simulink model "MultipleAgentsChoice_NoVR"  (Simulink 7.5)
settings: Solver=ode45  StartTime=0.0  StopTime=1000  RelTol=1e-4  AbsTol=1e-4
libraries: simulink x64
(part 3 of 6)

== system MultipleAgentsChoice_NoVR/StatePropagation/SatelliteControlAccel/Agent Body1/Actual Thruster response ==
  note: RELIABLE THRUSTER?
  Signals : Inport  OutDataType=sfix(16)  OutScaling=2^0
  AgentNumber : Inport  Port=2  OutDataType=sfix(16)  OutScaling=2^0
  Bus Creator{,1..3} (4 alike) : BusCreator  Inputs=3
  Bus Creator4 : BusCreator
  Bus Selector : BusSelector  OutputSignals=A1ControlSignals,ConfigurationSignals.XValves1,ConfigurationSignals.XSwitch1,ConfigurationSignals.YValves,ConfigurationSignals.YSwitch,ConfigurationSignals.ZValves,ConfigurationSignals.ZSwitch,ConfigurationSignals.XYZValves,ConfigurationSignals.XYZSwitch,ConfigurationSignals.A1Break
  Bus Selector1 : BusSelector  OutputSignals=signal1.L1Vent,signal1.L2Vent,signal2.L1Vent,signal2.L2Vent,signal3.L1Vent,signal3.L2Vent,XYZ.L1Vent,XYZ.L2Vent  OutputAsBus=on
  Constant{,1..3} (4 alike) : Constant  OutDataType=sfix(16)  OutScaling=2^0
  Conv2XYZ : MATLABFcn  MATLABFcn=Conv2XYZ_multi  OutputDimensions=3
  Demux : Demux
  Derivative : Derivative
  Mux : Mux  Inputs=5
  Mux1 : Mux  Inputs=2
  PressureTank : Subsystem
  Reliable : Constant  OutDataType=sfix(16)  OutScaling=2^0
  Sum : Sum  Inputs=|++  OutDataType=sfix(16)  OutScaling=2^0
  Switch : simulink/Signal Routing/Manual Switch  SystemSampleTime=-1  sw=1  action=0  varsize=off
  ThrusterSuiteNumber1 : Constant  Value=4  OutDataType=sfix(16)  OutScaling=2^0
  Unreliable : Constant  Value=0  OutDataType=sfix(16)  OutScaling=2^0
  VentForce : MATLABFcn  MATLABFcn=VentForce_multi  OutputDimensions=3
  XYZthruster : Subsystem
  Xthruster : Subsystem
  Ythruster1 : Subsystem
  Zthruster1 : Subsystem
  XThrusterData : Outport  OutDataType=sfix(16)  OutScaling=2^0
  YThrusterData : Outport  Port=2  OutDataType=sfix(16)  OutScaling=2^0
  ZThrusterData : Outport  Port=3  OutDataType=sfix(16)  OutScaling=2^0
  XYZThrusterData : Outport  Port=4  OutDataType=sfix(16)  OutScaling=2^0
  Forces : Outport  Port=5  OutDataType=sfix(16)  OutScaling=2^0
  PressureData : Outport  Port=6  OutDataType=sfix(16)  OutScaling=2^0
  wires:
  Bus Selector/9 -> Bus Creator3/3  "<XYZSwitch>"
  Bus Selector/8 -> Bus Creator3/2  "<XYZValves>"
  Bus Creator3/1 -> XYZthruster/3(Data)
  Constant2/1 -> Bus Creator3/1
  Demux/4 -> XYZthruster/2(ForceRequest)
  XYZthruster/2(XYZforces) -> Mux/4
  XYZthruster/1(XYZData) -> XYZThrusterData/1  "A1XYZThrusterData"
  Bus Selector/4 -> Bus Creator1/2  "<YValves>"
  Zthruster1/2(Zforces) -> Mux/3
  Bus Creator2/1 -> Zthruster1/3(Data)
  Constant1/1 -> Bus Creator2/1
  Bus Creator1/1 -> Ythruster1/3(Data)
  Constant/1 -> Bus Creator1/1
  Bus Selector/3 -> Bus Creator/3  "<XSwitch1>"
  Bus Selector/2 -> Bus Creator/2  "<XValves1>"
  Bus Creator/1 -> Xthruster/3(Data)
  Zthruster1/1(ZData) -> ZThrusterData/1  "A1ZThrusterData"
  Ythruster1/1(YData) -> YThrusterData/1  "A1YThrusterData"
  Xthruster/1(XData) -> XThrusterData/1
  Ythruster1/2(Yforces) -> Mux/2
  Demux/3 -> Zthruster1/2(ForceRequest)
  Demux/2 -> Ythruster1/2(ForceRequest)
  Bus Selector/7 -> Bus Creator2/3  "<ZSwitch>"
  Bus Selector/6 -> Bus Creator2/2  "<ZValves>"
  Bus Selector/5 -> Bus Creator1/3  "<YSwitch>"
  Xthruster/2(Xforces) -> Mux/1
  Demux/1 -> Xthruster/2(ForceRequest)
  Bus Selector/1 -> Demux/1  "<A1ControlSignals>"
  Mux/1 -> Conv2XYZ/1
  Signals/1 -> Bus Selector/1
  Constant3/1 -> Bus Creator/1
  AgentNumber/1 -> Mux/5
  Mux1/1 -> PressureData/1
  Bus Creator4/1 -> PressureTank/2(GroupVentData), Bus Selector1/1
  PressureTank/1(TankPressure) -> [FeedPressure], Derivative/1, Mux1/1  "MainTankPressure"
  ThrusterSuiteNumber1/1 -> [NumThrusters]
  [VentY] -> Bus Creator4/2
  [VentZ] -> Bus Creator4/3
  [VentXYZ] -> Bus Creator4/4
  [VentX] -> Bus Creator4/1
  Xthruster/3(ActivityData) -> [VentX]
  XYZthruster/3(Activitydata) -> [VentXYZ]
  Zthruster1/3(Activitydata) -> [VentZ]
  Ythruster1/3(ActivityData) -> [VentY]
  [FeedPressure] -> Xthruster/1(FeedPressure)
  [FeedPressure] -> Ythruster1/1(FeedPressure)
  [FeedPressure] -> Zthruster1/1(FeedPressure)
  [FeedPressure] -> XYZthruster/1(FeedPressure)
  [NumThrusters] -> PressureTank/1(NumThrusters)
  Derivative/1 -> Mux1/2  "MainTankDerrivative"
  Switch/1 -> Zthruster1/4(Reliability)
  Reliable/1 -> Switch/1
  Unreliable/1 -> Switch/2
  Bus Selector/10 -> Zthruster1/5(BrokenLine)  "<A1Break>"
  Conv2XYZ/1 -> Sum/2
  VentForce/1 -> Sum/1
  Sum/1 -> Forces/1
  Bus Selector1/1 -> VentForce/1

== system MultipleAgentsChoice_NoVR/StatePropagation/SatelliteControlAccel/Agent Body1/Convert2Accels ==
  note: convert forces to accelerations based on 20kg mass and conv to km units
  Forces : Inport  OutDataType=sfix(16)  OutScaling=2^0
  Conv KM : Gain  Gain=0.001  ParameterDataType=sfix(16)  ParameterScaling=2^0  OutDataType=sfix(16)  OutScaling=2^0
  mass : Gain  Gain=0.05  ParameterDataType=sfix(16)  ParameterScaling=2^0  OutDataType=sfix(16)  OutScaling=2^0
  Accels : Outport  OutDataType=sfix(16)  OutScaling=2^0
  wires:
  Forces/1 -> mass/1
  Conv KM/1 -> Accels/1
  mass/1 -> Conv KM/1

== system MultipleAgentsChoice_NoVR/StatePropagation/SatelliteControlAccel/Agent Body2/Actual Thruster response ==
  note: UNRELIABLE THRUSTER?
  Signals : Inport  OutDataType=sfix(16)  OutScaling=2^0
  AgentNumber : Inport  Port=2  OutDataType=sfix(16)  OutScaling=2^0
  Bus Creator{,1..3} (4 alike) : BusCreator  Inputs=3
  Bus Creator4 : BusCreator
  Bus Selector : BusSelector  OutputSignals=A2ControlSignals,ConfigurationSignals.XValves1,ConfigurationSignals.XSwitch1,ConfigurationSignals.YValves,ConfigurationSignals.YSwitch,ConfigurationSignals.ZValves,ConfigurationSignals.ZSwitch,ConfigurationSignals.XYZValves,ConfigurationSignals.XYZSwitch,ConfigurationSignals.A2Break
  Bus Selector1 : BusSelector  OutputSignals=signal1.L1Vent,signal1.L2Vent,signal2.L1Vent,signal2.L2Vent,signal3.L1Vent,signal3.L2Vent,XYZ.L1Vent,XYZ.L2Vent  OutputAsBus=on
  Constant{,1..3} (4 alike) : Constant  OutDataType=sfix(16)  OutScaling=2^0
  Conv2XYZ : MATLABFcn  MATLABFcn=Conv2XYZ_multi  OutputDimensions=3
  Demux : Demux
  Derivative : Derivative
  Mux : Mux  Inputs=5
  Mux1 : Mux  Inputs=2
  PressureTank : Subsystem
  Reliable : Constant  OutDataType=sfix(16)  OutScaling=2^0
  Sum : Sum  Inputs=|++  OutDataType=sfix(16)  OutScaling=2^0
  Switch : simulink/Signal Routing/Manual Switch  SystemSampleTime=-1  sw=1  action=0  varsize=off
  ThrusterSuiteNumber1 : Constant  Value=4  OutDataType=sfix(16)  OutScaling=2^0
  Unreliable : Constant  Value=0  OutDataType=sfix(16)  OutScaling=2^0
  VentForce : MATLABFcn  MATLABFcn=VentForce_multi  OutputDimensions=3
  XYZthruster : Subsystem
  Xthruster : Subsystem
  Ythruster1 : Subsystem
  Zthruster1 : Subsystem
  XThrusterData : Outport  OutDataType=sfix(16)  OutScaling=2^0
  YThrusterData : Outport  Port=2  OutDataType=sfix(16)  OutScaling=2^0
  ZThrusterData : Outport  Port=3  OutDataType=sfix(16)  OutScaling=2^0
  XYZThrusterData : Outport  Port=4  OutDataType=sfix(16)  OutScaling=2^0
  Forces : Outport  Port=5  OutDataType=sfix(16)  OutScaling=2^0
  PressureData : Outport  Port=6  OutDataType=sfix(16)  OutScaling=2^0
  wires:
  Derivative/1 -> Mux1/2  "MainTankDerrivative"
  [NumThrusters] -> PressureTank/1(NumThrusters)
  [FeedPressure] -> XYZthruster/1(FeedPressure)
  [FeedPressure] -> Zthruster1/1(FeedPressure)
  [FeedPressure] -> Ythruster1/1(FeedPressure)
  [FeedPressure] -> Xthruster/1(FeedPressure)
  Ythruster1/3(ActivityData) -> [VentY]
  Zthruster1/3(Activitydata) -> [VentZ]
  XYZthruster/3(Activitydata) -> [VentXYZ]
  Xthruster/3(ActivityData) -> [VentX]
  [VentX] -> Bus Creator4/1
  [VentXYZ] -> Bus Creator4/4
  [VentZ] -> Bus Creator4/3
  [VentY] -> Bus Creator4/2
  ThrusterSuiteNumber1/1 -> [NumThrusters]
  PressureTank/1(TankPressure) -> Mux1/1, Derivative/1, [FeedPressure]  "MainTankPressure"
  Bus Creator4/1 -> PressureTank/2(GroupVentData), Bus Selector1/1
  Mux1/1 -> PressureData/1
  AgentNumber/1 -> Mux/5
  Constant3/1 -> Bus Creator/1
  Signals/1 -> Bus Selector/1
  Mux/1 -> Conv2XYZ/1
  Bus Selector/1 -> Demux/1  "<A2ControlSignals>"
  Demux/1 -> Xthruster/2(ForceRequest)
  Xthruster/2(Xforces) -> Mux/1
  Bus Selector/5 -> Bus Creator1/3  "<YSwitch>"
  Bus Selector/6 -> Bus Creator2/2  "<ZValves>"
  Bus Selector/7 -> Bus Creator2/3  "<ZSwitch>"
  Demux/2 -> Ythruster1/2(ForceRequest)
  Demux/3 -> Zthruster1/2(ForceRequest)
  Ythruster1/2(Yforces) -> Mux/2
  Xthruster/1(XData) -> XThrusterData/1  "A2XThrusterData"
  Ythruster1/1(YData) -> YThrusterData/1  "A2YThrusterData"
  Zthruster1/1(ZData) -> ZThrusterData/1  "A2ZThrusterData"
  Bus Creator/1 -> Xthruster/3(Data)
  Bus Selector/2 -> Bus Creator/2  "<XValves1>"
  Bus Selector/3 -> Bus Creator/3  "<XSwitch1>"
  Constant/1 -> Bus Creator1/1
  Bus Creator1/1 -> Ythruster1/3(Data)
  Constant1/1 -> Bus Creator2/1
  Bus Creator2/1 -> Zthruster1/3(Data)
  Zthruster1/2(Zforces) -> Mux/3
  Bus Selector/4 -> Bus Creator1/2  "<YValves>"
  XYZthruster/1(XYZData) -> XYZThrusterData/1  "A2XYZThrusterData"
  XYZthruster/2(XYZforces) -> Mux/4
  Demux/4 -> XYZthruster/2(ForceRequest)
  Constant2/1 -> Bus Creator3/1
  Bus Creator3/1 -> XYZthruster/3(Data)
  Bus Selector/8 -> Bus Creator3/2  "<XYZValves>"
  Bus Selector/9 -> Bus Creator3/3  "<XYZSwitch>"
  Unreliable/1 -> Switch/2
  Reliable/1 -> Switch/1
  Switch/1 -> Zthruster1/4(Reliability)
  Bus Selector/10 -> Zthruster1/5(BrokenLine)  "<A2Break>"
  VentForce/1 -> Sum/1
  Sum/1 -> Forces/1
  Conv2XYZ/1 -> Sum/2
  Bus Selector1/1 -> VentForce/1

== system MultipleAgentsChoice_NoVR/StatePropagation/SatelliteControlAccel/Agent Body2/Convert2Accels ==
  note: convert forces to accelerations based on 20kg mass and conv to km units
  Forces : Inport  OutDataType=sfix(16)  OutScaling=2^0
  Conv KM : Gain  Gain=0.001  ParameterDataType=sfix(16)  ParameterScaling=2^0  OutDataType=sfix(16)  OutScaling=2^0
  mass : Gain  Gain=0.05  ParameterDataType=sfix(16)  ParameterScaling=2^0  OutDataType=sfix(16)  OutScaling=2^0
  Accels : Outport  OutDataType=sfix(16)  OutScaling=2^0
  wires:
  mass/1 -> Conv KM/1
  Conv KM/1 -> Accels/1
  Forces/1 -> mass/1

== system MultipleAgentsChoice_NoVR/StatePropagation/SatelliteControlAccel/Agent Body3/Actual Thruster response ==
  note: UNRELIABLE THRUSTER?
  Signals : Inport  OutDataType=sfix(16)  OutScaling=2^0
  AgentNumber : Inport  Port=2  OutDataType=sfix(16)  OutScaling=2^0
  Bus Creator{,1..3} (4 alike) : BusCreator  Inputs=3
  Bus Creator4 : BusCreator
  Bus Selector : BusSelector  OutputSignals=A3ControlSignals,ConfigurationSignals.XValves1,ConfigurationSignals.XSwitch1,ConfigurationSignals.YValves,ConfigurationSignals.YSwitch,ConfigurationSignals.ZValves,ConfigurationSignals.ZSwitch,ConfigurationSignals.XYZValves,ConfigurationSignals.XYZSwitch,ConfigurationSignals.A3Break
  Bus Selector1 : BusSelector  OutputSignals=signal1.L1Vent,signal1.L2Vent,signal2.L1Vent,signal2.L2Vent,signal3.L1Vent,signal3.L2Vent,XYZ.L1Vent,XYZ.L2Vent  OutputAsBus=on
  Constant{,1..3} (4 alike) : Constant  OutDataType=sfix(16)  OutScaling=2^0
  Conv2XYZ : MATLABFcn  MATLABFcn=Conv2XYZ_multi  OutputDimensions=3
  Demux : Demux
  Derivative : Derivative
  Mux : Mux  Inputs=5
  Mux1 : Mux  Inputs=2
  PressureTank : Subsystem
  Reliable : Constant  OutDataType=sfix(16)  OutScaling=2^0
  Sum : Sum  Inputs=|++  OutDataType=sfix(16)  OutScaling=2^0
  Switch : simulink/Signal Routing/Manual Switch  SystemSampleTime=-1  sw=1  action=0  varsize=off
  ThrusterSuiteNumber1 : Constant  Value=4  OutDataType=sfix(16)  OutScaling=2^0
  Unreliable : Constant  Value=0  OutDataType=sfix(16)  OutScaling=2^0
  VentForce : MATLABFcn  MATLABFcn=VentForce_multi  OutputDimensions=3
  XYZthruster : Subsystem
  Xthruster : Subsystem
  Ythruster1 : Subsystem
  Zthruster1 : Subsystem
  XThrusterData : Outport  OutDataType=sfix(16)  OutScaling=2^0
  YThrusterData : Outport  Port=2  OutDataType=sfix(16)  OutScaling=2^0
  ZThrusterData : Outport  Port=3  OutDataType=sfix(16)  OutScaling=2^0
  XYZThrusterData : Outport  Port=4  OutDataType=sfix(16)  OutScaling=2^0
  Forces : Outport  Port=5  OutDataType=sfix(16)  OutScaling=2^0
  PressureData : Outport  Port=6  OutDataType=sfix(16)  OutScaling=2^0
  wires:
  Derivative/1 -> Mux1/2  "MainTankDerrivative"
  [NumThrusters] -> PressureTank/1(NumThrusters)
  [FeedPressure] -> XYZthruster/1(FeedPressure)
  [FeedPressure] -> Zthruster1/1(FeedPressure)
  [FeedPressure] -> Ythruster1/1(FeedPressure)
  [FeedPressure] -> Xthruster/1(FeedPressure)
  Ythruster1/3(ActivityData) -> [VentY]
  Zthruster1/3(Activitydata) -> [VentZ]
  XYZthruster/3(Activitydata) -> [VentXYZ]
  Xthruster/3(ActivityData) -> [VentX]
  [VentX] -> Bus Creator4/1
  [VentXYZ] -> Bus Creator4/4
  [VentZ] -> Bus Creator4/3
  [VentY] -> Bus Creator4/2
  ThrusterSuiteNumber1/1 -> [NumThrusters]
  PressureTank/1(TankPressure) -> Mux1/1, Derivative/1, [FeedPressure]  "MainTankPressure"
  Bus Creator4/1 -> PressureTank/2(GroupVentData), Bus Selector1/1
  Mux1/1 -> PressureData/1
  AgentNumber/1 -> Mux/5
  Constant3/1 -> Bus Creator/1
  Signals/1 -> Bus Selector/1
  Mux/1 -> Conv2XYZ/1
  Bus Selector/1 -> Demux/1  "<A3ControlSignals>"
  Demux/1 -> Xthruster/2(ForceRequest)
  Xthruster/2(Xforces) -> Mux/1
  Bus Selector/5 -> Bus Creator1/3  "<YSwitch>"
  Bus Selector/6 -> Bus Creator2/2  "<ZValves>"
  Bus Selector/7 -> Bus Creator2/3  "<ZSwitch>"
  Demux/2 -> Ythruster1/2(ForceRequest)
  Demux/3 -> Zthruster1/2(ForceRequest)
  Ythruster1/2(Yforces) -> Mux/2
  Xthruster/1(XData) -> XThrusterData/1  "A3XThrusterData"
  Ythruster1/1(YData) -> YThrusterData/1  "A3YThrusterData"
  Zthruster1/1(ZData) -> ZThrusterData/1  "A3ZThrusterData"
  Bus Creator/1 -> Xthruster/3(Data)
  Bus Selector/2 -> Bus Creator/2  "<XValves1>"
  Bus Selector/3 -> Bus Creator/3  "<XSwitch1>"
  Constant/1 -> Bus Creator1/1
  Bus Creator1/1 -> Ythruster1/3(Data)
  Constant1/1 -> Bus Creator2/1
  Bus Creator2/1 -> Zthruster1/3(Data)
  Zthruster1/2(Zforces) -> Mux/3
  Bus Selector/4 -> Bus Creator1/2  "<YValves>"
  XYZthruster/1(XYZData) -> XYZThrusterData/1  "A3XYZThrusterData"
  XYZthruster/2(XYZforces) -> Mux/4
  Demux/4 -> XYZthruster/2(ForceRequest)
  Constant2/1 -> Bus Creator3/1
  Bus Creator3/1 -> XYZthruster/3(Data)
  Bus Selector/8 -> Bus Creator3/2  "<XYZValves>"
  Bus Selector/9 -> Bus Creator3/3  "<XYZSwitch>"
  Unreliable/1 -> Switch/2
  Reliable/1 -> Switch/1
  Switch/1 -> Zthruster1/4(Reliability)
  Bus Selector/10 -> Zthruster1/5(BrokenLine)  "<A3Break>"
  VentForce/1 -> Sum/1
  Sum/1 -> Forces/1
  Conv2XYZ/1 -> Sum/2
  Bus Selector1/1 -> VentForce/1

== system MultipleAgentsChoice_NoVR/StatePropagation/SatelliteControlAccel/Agent Body3/Convert2Accels ==
  note: convert forces to accelerations based on 20kg mass and conv to km units
  Forces : Inport  OutDataType=sfix(16)  OutScaling=2^0
  Conv KM : Gain  Gain=0.001  ParameterDataType=sfix(16)  ParameterScaling=2^0  OutDataType=sfix(16)  OutScaling=2^0
  mass : Gain  Gain=0.05  ParameterDataType=sfix(16)  ParameterScaling=2^0  OutDataType=sfix(16)  OutScaling=2^0
  Accels : Outport  OutDataType=sfix(16)  OutScaling=2^0
  wires:
  Forces/1 -> mass/1
  Conv KM/1 -> Accels/1
  mass/1 -> Conv KM/1

== system MultipleAgentsChoice_NoVR/StatePropagation/SatelliteControlAccel/GetCmdAIL/Triggered run ==
  Trigger : TriggerPort
  DimentionsOut1 : Constant  Value=127  OutDataType=sfix(16)  OutScaling=2^0
  GetCmdAILXYZ : MATLABFcn  MATLABFcn=GetCmdAIL  OutputDimensions=127
  Commands : Outport  OutDataType=sfix(16)  OutScaling=2^0
  wires:
  DimentionsOut1/1 -> GetCmdAILXYZ/1
  GetCmdAILXYZ/1 -> Commands/1

== system MultipleAgentsChoice_NoVR/StatePropagation/SatelliteControlAccel/Selective Hill State Provision and Discretisation/Agent1 ==
  GEOC_Current : Inport  OutDataType=sfix(16)  OutScaling=2^0
  LeadAgent : Inport  Port=2  OutDataType=sfix(16)  OutScaling=2^0
  Bus Creator : BusCreator  Inputs=5
  Bus Selector2 : BusSelector  OutputSignals=Agent1Pos,Agent1Vel,Agent2Pos,Agent2Vel,Agent3Pos,Agent3Vel
  Demux : Demux  Outputs=7
  Hill State multi : MATLABFcn  MATLABFcn=HillErrors_multi  OutputDimensions=7
  Multiport Switch : MultiPortSwitch  zeroidx=off
  Mux1 : Mux  Inputs=3
  Mux2 : Mux  Inputs=3
  Mux{3..6} (4 alike) : Mux  Inputs=2
  Zero-Order Hold3 : ZeroOrderHold  SampleTime=0.5
  Zero-Order Hold4 : ZeroOrderHold  SampleTime=0.5
  Agent1 : Outport  OutDataType=sfix(16)  OutScaling=2^0
  wires:
  Mux1/1 -> Zero-Order Hold4/1, Bus Creator/3  "HillVelCont"
  Mux2/1 -> Zero-Order Hold3/1, Bus Creator/2  "HillPosCont"
  Demux/2 -> Mux2/1
  Demux/4 -> Mux2/3
  Demux/3 -> Mux2/2
  Demux/7 -> Mux1/3
  Demux/5 -> Mux1/1
  Demux/6 -> Mux1/2
  Hill State multi/1 -> Demux/1
  LeadAgent/1 -> Multiport Switch/1
  GEOC_Current/1 -> Bus Selector2/1
  Demux/1 -> Bus Creator/1  "HillMagCont"
  Bus Creator/1 -> Agent1/1  "A1HillState"
  Mux3/1 -> Hill State multi/1
  Bus Selector2/1 -> Mux4/1  "<Agent1Pos>"
  Bus Selector2/2 -> Mux4/2  "<Agent1Vel>"
  Bus Selector2/3 -> Mux5/1  "<Agent2Pos>"
  Bus Selector2/4 -> Mux5/2  "<Agent2Vel>"
  Bus Selector2/5 -> Mux6/1  "<Agent3Pos>"
  Bus Selector2/6 -> Mux6/2  "<Agent3Vel>"
  Mux4/1 -> [Agent1]
  Mux5/1 -> [Agent2]
  Mux6/1 -> [Agent3]
  Multiport Switch/1 -> Mux3/2
  [Agent1] -> Multiport Switch/2
  [Agent2] -> Multiport Switch/3
  [Agent3] -> Multiport Switch/4
  [Agent1] -> Mux3/1
  Zero-Order Hold4/1 -> Bus Creator/5  "HillVelDisc"
  Zero-Order Hold3/1 -> Bus Creator/4  "HillPosDisc"

== system MultipleAgentsChoice_NoVR/StatePropagation/SatelliteControlAccel/Selective Hill State Provision and Discretisation/Agent2 ==
  GEOC_Current : Inport  OutDataType=sfix(16)  OutScaling=2^0
  LeadAgent : Inport  Port=2  OutDataType=sfix(16)  OutScaling=2^0
  Bus Creator : BusCreator  Inputs=5
  Bus Selector2 : BusSelector  OutputSignals=Agent1Pos,Agent1Vel,Agent2Pos,Agent2Vel,Agent3Pos,Agent3Vel
  Demux : Demux  Outputs=7
  Hill State multi : MATLABFcn  MATLABFcn=HillErrors_multi  OutputDimensions=7
  Multiport Switch : MultiPortSwitch  zeroidx=off
  Mux1 : Mux  Inputs=3
  Mux2 : Mux  Inputs=3
  Mux{3..6} (4 alike) : Mux  Inputs=2
  Zero-Order Hold3 : ZeroOrderHold  SampleTime=0.5
  Zero-Order Hold4 : ZeroOrderHold  SampleTime=0.5
  Agent2 : Outport  OutDataType=sfix(16)  OutScaling=2^0
  wires:
  [Agent3] -> Multiport Switch/4
  [Agent2] -> Multiport Switch/3
  [Agent1] -> Multiport Switch/2
  Multiport Switch/1 -> Mux3/2
  Mux6/1 -> [Agent3]
  Mux5/1 -> [Agent2]
  Mux4/1 -> [Agent1]
  Bus Selector2/6 -> Mux6/2  "<Agent3Vel>"
  Bus Selector2/5 -> Mux6/1  "<Agent3Pos>"
  Bus Selector2/4 -> Mux5/2  "<Agent2Vel>"
  Bus Selector2/3 -> Mux5/1  "<Agent2Pos>"
  Bus Selector2/2 -> Mux4/2  "<Agent1Vel>"
  Bus Selector2/1 -> Mux4/1  "<Agent1Pos>"
  [Agent2] -> Mux3/1
  Mux3/1 -> Hill State multi/1
  Bus Creator/1 -> Agent2/1  "A2HillState"
  Demux/1 -> Bus Creator/1  "HillMagCont"
  GEOC_Current/1 -> Bus Selector2/1
  LeadAgent/1 -> Multiport Switch/1
  Hill State multi/1 -> Demux/1
  Demux/6 -> Mux1/2
  Demux/5 -> Mux1/1
  Demux/7 -> Mux1/3
  Demux/3 -> Mux2/2
  Demux/4 -> Mux2/3
  Demux/2 -> Mux2/1
  Mux2/1 -> Zero-Order Hold3/1, Bus Creator/2  "HillPosCont"
  Mux1/1 -> Zero-Order Hold4/1, Bus Creator/3  "HillVelCont"
  Zero-Order Hold3/1 -> Bus Creator/4  "HillPosDisc"
  Zero-Order Hold4/1 -> Bus Creator/5  "HillVelDisc"

== system MultipleAgentsChoice_NoVR/StatePropagation/SatelliteControlAccel/Selective Hill State Provision and Discretisation/Agent3 ==
  GEOC_Current : Inport  OutDataType=sfix(16)  OutScaling=2^0
  LeadAgent : Inport  Port=2  OutDataType=sfix(16)  OutScaling=2^0
  Bus Creator : BusCreator  Inputs=5
  Bus Selector2 : BusSelector  OutputSignals=Agent1Pos,Agent1Vel,Agent2Pos,Agent2Vel,Agent3Pos,Agent3Vel
  Demux : Demux  Outputs=7
  Hill State multi : MATLABFcn  MATLABFcn=HillErrors_multi  OutputDimensions=7
  Multiport Switch : MultiPortSwitch  zeroidx=off
  Mux1 : Mux  Inputs=3
  Mux2 : Mux  Inputs=3
  Mux{3..6} (4 alike) : Mux  Inputs=2
  Zero-Order Hold3 : ZeroOrderHold  SampleTime=0.5
  Zero-Order Hold4 : ZeroOrderHold  SampleTime=0.5
  Agent3 : Outport  OutDataType=sfix(16)  OutScaling=2^0
  wires:
  Mux1/1 -> Zero-Order Hold4/1, Bus Creator/3  "HillVelCont"
  Mux2/1 -> Zero-Order Hold3/1, Bus Creator/2  "HillPosCont"
  Demux/2 -> Mux2/1
  Demux/4 -> Mux2/3
  Demux/3 -> Mux2/2
  Demux/7 -> Mux1/3
  Demux/5 -> Mux1/1
  Demux/6 -> Mux1/2
  Hill State multi/1 -> Demux/1
  LeadAgent/1 -> Multiport Switch/1
  GEOC_Current/1 -> Bus Selector2/1
  Zero-Order Hold4/1 -> Bus Creator/5  "HillVelDisc"
  Demux/1 -> Bus Creator/1  "HillMagCont"
  Bus Creator/1 -> Agent3/1  "A3HillState"
  Mux3/1 -> Hill State multi/1
  Bus Selector2/1 -> Mux4/1  "<Agent1Pos>"
  Bus Selector2/2 -> Mux4/2  "<Agent1Vel>"
  Bus Selector2/3 -> Mux5/1  "<Agent2Pos>"
  Bus Selector2/4 -> Mux5/2  "<Agent2Vel>"
  Bus Selector2/5 -> Mux6/1  "<Agent3Pos>"
  Bus Selector2/6 -> Mux6/2  "<Agent3Vel>"
  Mux4/1 -> [Agent1]
  Mux5/1 -> [Agent2]
  Mux6/1 -> [Agent3]
  [Agent1] -> Multiport Switch/2
  [Agent2] -> Multiport Switch/3
  [Agent3] -> Multiport Switch/4
  [Agent3] -> Mux3/1
  Multiport Switch/1 -> Mux3/2
  Zero-Order Hold3/1 -> Bus Creator/4  "HillPosDisc"

== system MultipleAgentsChoice_NoVR/StatePropagation/SatelliteControlAccel/Selective Hill State Provision and Discretisation/MemoryUpdate ==
  GEOC_Current : Inport  OutDataType=sfix(16)  OutScaling=2^0
  LeadAgent : Inport  Port=2  OutDataType=sfix(16)  OutScaling=2^0
  Bus Selector2 : BusSelector  OutputSignals=Agent1Pos,Agent1Vel,Agent2Pos,Agent2Vel,Agent3Pos,Agent3Vel
  Multiport Switch : MultiPortSwitch  zeroidx=off
  Mux4 : Mux  Inputs=2
  Mux5 : Mux  Inputs=2
  Mux6 : Mux  Inputs=2
  Updatememory : MATLABFcn  MATLABFcn=UpdateMemory  OutputDimensions=0
  wires:
  Multiport Switch/1 -> Updatememory/1
  Mux6/1 -> Multiport Switch/4
  Mux5/1 -> Multiport Switch/3
  Mux4/1 -> Multiport Switch/2
  Bus Selector2/6 -> Mux6/2  "<Agent3Vel>"
  Bus Selector2/5 -> Mux6/1  "<Agent3Pos>"
  Bus Selector2/4 -> Mux5/2  "<Agent2Vel>"
  Bus Selector2/3 -> Mux5/1  "<Agent2Pos>"
  Bus Selector2/2 -> Mux4/2  "<Agent1Vel>"
  Bus Selector2/1 -> Mux4/1  "<Agent1Pos>"
  GEOC_Current/1 -> Bus Selector2/1
  LeadAgent/1 -> Multiport Switch/1

== system MultipleAgentsChoice_NoVR/StatePropagation/SatelliteControlAccel/TriggeredSendAgent/SendToAIL ==
  A1ActualForces : Inport  OutDataType=sfix(16)  OutScaling=2^0
  A1PlanMsg : Inport  Port=2  OutDataType=sfix(16)  OutScaling=2^0
  A1DesiredForces : Inport  Port=3  OutDataType=sfix(16)  OutScaling=2^0
  A1StateInfo : Inport  Port=4  OutDataType=sfix(16)  OutScaling=2^0
  A1tank : Inport  Port=5  OutDataType=sfix(16)  OutScaling=2^0
  A1XThruster : Inport  Port=6  OutDataType=sfix(16)  OutScaling=2^0
  A1YThruster : Inport  Port=7  OutDataType=sfix(16)  OutScaling=2^0
  A1ZThruster : Inport  Port=8  OutDataType=sfix(16)  OutScaling=2^0
  A1XYZThruster : Inport  Port=9  OutDataType=sfix(16)  OutScaling=2^0
  A2ActualForces : Inport  Port=10  OutDataType=sfix(16)  OutScaling=2^0
  A2PlanMsg : Inport  Port=11  OutDataType=sfix(16)  OutScaling=2^0
  A2DesiredForces : Inport  Port=12  OutDataType=sfix(16)  OutScaling=2^0
  A2StateInfo : Inport  Port=13  OutDataType=sfix(16)  OutScaling=2^0
  A2tank : Inport  Port=14  OutDataType=sfix(16)  OutScaling=2^0
  A2XThruster : Inport  Port=15  OutDataType=sfix(16)  OutScaling=2^0
  A2YThruster : Inport  Port=16  OutDataType=sfix(16)  OutScaling=2^0
  A2ZThruster : Inport  Port=17  OutDataType=sfix(16)  OutScaling=2^0
  A2XYZThruster : Inport  Port=18  OutDataType=sfix(16)  OutScaling=2^0
  A3ActualForces : Inport  Port=19  OutDataType=sfix(16)  OutScaling=2^0
  A3PlanMsg : Inport  Port=20  OutDataType=sfix(16)  OutScaling=2^0
  A3DesiredForces : Inport  Port=21  OutDataType=sfix(16)  OutScaling=2^0
  A3StateInfo : Inport  Port=22  OutDataType=sfix(16)  OutScaling=2^0
  A3tank : Inport  Port=23  OutDataType=sfix(16)  OutScaling=2^0
  A3XThruster : Inport  Port=24  OutDataType=sfix(16)  OutScaling=2^0
  A3YThruster : Inport  Port=25  OutDataType=sfix(16)  OutScaling=2^0
  A3ZThruster : Inport  Port=26  OutDataType=sfix(16)  OutScaling=2^0
  A3XYZThruster : Inport  Port=27  OutDataType=sfix(16)  OutScaling=2^0
  Display : Display
  MATLAB Fcn : MATLABFcn  MATLABFcn=CommunicateWithTagsMulti  OutputDimensions=0
  Mux : Mux  Inputs=27
  wires:
  A1ActualForces/1 -> Mux/1  "A1ActualForces"
  A1PlanMsg/1 -> Mux/2  "A1PlanMsg"
  A1StateInfo/1 -> Mux/4  "A1StateInfo"
  A1XThruster/1 -> Mux/6  "A1XThruster"
  A1YThruster/1 -> Mux/7  "A1YThruster"
  A1ZThruster/1 -> Mux/8  "A1ZThruster"
  A1DesiredForces/1 -> Mux/3  "A1DesiredForfces"
  A1tank/1 -> Mux/5  "A1Tank"
  A2ActualForces/1 -> Mux/10  "A2ActualForces"
  A2PlanMsg/1 -> Mux/11  "A2PlanMsg"
  A2StateInfo/1 -> Mux/13  "A2StateInfo"
  A2XThruster/1 -> Mux/15  "A2XThruster"
  A2YThruster/1 -> Mux/16  "A2YThruster"
  A2ZThruster/1 -> Mux/17  "A2ZThruster"
  A2DesiredForces/1 -> Mux/12  "A2DesiredForces"
  A2tank/1 -> Mux/14  "A2Tank"
  A1XYZThruster/1 -> Mux/9  "A1XYZThruster"
  A2XYZThruster/1 -> Mux/18  "A2XYZThruster"
  A3PlanMsg/1 -> Mux/20  "A3PlanMsg"
  A3DesiredForces/1 -> Mux/21  "A3DesiredForces"
  A3StateInfo/1 -> Mux/22  "A3StateInfo"
  A3tank/1 -> Mux/23  "A3Tank"
  A3XThruster/1 -> Mux/24  "A3XThruster"
  A3YThruster/1 -> Mux/25  "A3YThruster"
  A3ZThruster/1 -> Mux/26  "A3ZThruster"
  A3XYZThruster/1 -> Mux/27  "A3XYZThruster"
  A3ActualForces/1 -> Mux/19  "A3ActualForces"
  Mux/1 -> MATLAB Fcn/1, Display/1

== system MultipleAgentsChoice_NoVR/StatePropagation/SatelliteControlAccel/TriggeredSendCont/SendToCont ==
  A1ActualForces : Inport  OutDataType=sfix(16)  OutScaling=2^0
  A1PlanMsg : Inport  Port=2  OutDataType=sfix(16)  OutScaling=2^0
  A1DesiredForces : Inport  Port=3  OutDataType=sfix(16)  OutScaling=2^0
  A1StateInfo : Inport  Port=4  OutDataType=sfix(16)  OutScaling=2^0
  A1tank : Inport  Port=5  OutDataType=sfix(16)  OutScaling=2^0
  A1XThruster : Inport  Port=6  OutDataType=sfix(16)  OutScaling=2^0
  A1YThruster : Inport  Port=7  OutDataType=sfix(16)  OutScaling=2^0
  A1ZThruster : Inport  Port=8  OutDataType=sfix(16)  OutScaling=2^0
  A1XYZThruster : Inport  Port=9  OutDataType=sfix(16)  OutScaling=2^0
  A2ActualForces : Inport  Port=10  OutDataType=sfix(16)  OutScaling=2^0
  A2PlanMsg : Inport  Port=11  OutDataType=sfix(16)  OutScaling=2^0
  A2DesiredForces : Inport  Port=12  OutDataType=sfix(16)  OutScaling=2^0
  A2StateInfo : Inport  Port=13  OutDataType=sfix(16)  OutScaling=2^0
  A2tank : Inport  Port=14  OutDataType=sfix(16)  OutScaling=2^0
  A2XThruster : Inport  Port=15  OutDataType=sfix(16)  OutScaling=2^0
  A2YThruster : Inport  Port=16  OutDataType=sfix(16)  OutScaling=2^0
  A2ZThruster : Inport  Port=17  OutDataType=sfix(16)  OutScaling=2^0
  A2XYZThruster : Inport  Port=18  OutDataType=sfix(16)  OutScaling=2^0
  A3ActualForces : Inport  Port=19  OutDataType=sfix(16)  OutScaling=2^0
  A3PlanMsg : Inport  Port=20  OutDataType=sfix(16)  OutScaling=2^0
  A3DesiredForces : Inport  Port=21  OutDataType=sfix(16)  OutScaling=2^0
  A3StateInfo : Inport  Port=22  OutDataType=sfix(16)  OutScaling=2^0
  A3tank : Inport  Port=23  OutDataType=sfix(16)  OutScaling=2^0
  A3XThruster : Inport  Port=24  OutDataType=sfix(16)  OutScaling=2^0
  A3YThruster : Inport  Port=25  OutDataType=sfix(16)  OutScaling=2^0
  A3ZThruster : Inport  Port=26  OutDataType=sfix(16)  OutScaling=2^0
  A3XYZThruster : Inport  Port=27  OutDataType=sfix(16)  OutScaling=2^0
  Display : Display
  MATLAB Fcn : MATLABFcn  MATLABFcn=CommunicateWithCont  OutputDimensions=0
  Mux : Mux  Inputs=27
  wires:
  Mux/1 -> Display/1, MATLAB Fcn/1
  A3ActualForces/1 -> Mux/19  "A3ActualForces"
  A3XYZThruster/1 -> Mux/27  "A3XYZThruster"
  A3ZThruster/1 -> Mux/26  "A3ZThruster"
  A3YThruster/1 -> Mux/25  "A3YThruster"
  A3XThruster/1 -> Mux/24  "A3XThruster"
  A3tank/1 -> Mux/23  "A3tank"
  A3StateInfo/1 -> Mux/22  "A3StateInfo"
  A3DesiredForces/1 -> Mux/21  "A3DesiredForces"
  A3PlanMsg/1 -> Mux/20  "A3PlanMsg"
  A2XYZThruster/1 -> Mux/18  "A2XYZThruster"
  A1XYZThruster/1 -> Mux/9  "A1XYZThruster"
  A2tank/1 -> Mux/14  "A2tank"
  A2DesiredForces/1 -> Mux/12  "A2DesiredForces"
  A2ZThruster/1 -> Mux/17  "A2ZThruster"
  A2YThruster/1 -> Mux/16  "A2YThruster"
  A2XThruster/1 -> Mux/15  "A2XThruster"
  A2StateInfo/1 -> Mux/13  "A2StateInfo"
  A2PlanMsg/1 -> Mux/11  "A2PlanMsg"
  A2ActualForces/1 -> Mux/10  "A2ActualForces"
  A1tank/1 -> Mux/5  "A1tank"
  A1DesiredForces/1 -> Mux/3  "A1DesiredForfces"
  A1ZThruster/1 -> Mux/8  "A1ZThruster"
  A1YThruster/1 -> Mux/7  "A1YThruster"
  A1XThruster/1 -> Mux/6  "A1XThruster"
  A1StateInfo/1 -> Mux/4  "A1StateInfo"
  A1PlanMsg/1 -> Mux/2  "A1PlanMsg"
  A1ActualForces/1 -> Mux/1  "A1ActualForces"

== system MultipleAgentsChoice_NoVR/StatePropagation/SatelliteControlAccel/Agent Body1/Actual Thruster response/PressureTank ==
  NumThrusters : Inport  OutDataType=sfix(16)  OutScaling=2^0
  GroupVentData : Inport  Port=2  OutDataType=sfix(16)  OutScaling=2^0
  Clock : Clock
      settings: Decimation=10
  Display : Display
  DropRate : MATLABFcn  MATLABFcn=DropRate_multi  OutputDimensions=1
  Integrator : Integrator  InitialConditionSource=external
  Mux : Mux  Inputs=2
  Start : Constant  Value=0  OutDataType=sfix(16)  OutScaling=2^0
  StartPressure : Constant  Value=100  OutDataType=sfix(16)  OutScaling=2^0
  Switch1 : Switch
  TankPressure : Outport  OutDataType=sfix(16)  OutScaling=2^0
  wires:
  DropRate/1 -> Switch1/1
  Mux/1 -> DropRate/1
  NumThrusters/1 -> Mux/1
  GroupVentData/1 -> Mux/2
  Switch1/1 -> Integrator/1
  Clock/1 -> Switch1/2
  Start/1 -> Switch1/3
  Integrator/1 -> Display/1, TankPressure/1
  StartPressure/1 -> Integrator/2

== system MultipleAgentsChoice_NoVR/StatePropagation/SatelliteControlAccel/Agent Body1/Actual Thruster response/XYZthruster ==
  note: NB:-Agent has no knowledge of red blocks
      |             -Blue blocks prescribed by agent
  note: Tank pressure and thruster selection: must declare number of thrusters
  FeedPressure : Inport  OutDataType=sfix(16)  OutScaling=2^0
  ForceRequest : Inport  Port=2  OutDataType=sfix(16)  OutScaling=2^0
  Data : Inport  Port=3  OutDataType=sfix(16)  OutScaling=2^0
  Bus Creator2 : BusCreator  Inputs=3
  Bus Selector : BusSelector  OutputSignals=XYZValves,XYZSwitch
  Constant : Constant  OutDataType=sfix(16)  OutScaling=2^0
  Constant1 : Constant  Value=0  OutDataType=sfix(16)  OutScaling=2^0
  Switch : Switch  Criteria=u2 ~= 0
  Thruster1 : Subsystem
  XYZData : Outport  OutDataType=sfix(16)  OutScaling=2^0
  XYZforces : Outport  Port=2  OutDataType=sfix(16)  OutScaling=2^0
  Activitydata : Outport  Port=3  OutDataType=sfix(16)  OutScaling=2^0
  wires:
  ForceRequest/1 -> Thruster1/4(ForceRequest)  "XYZforces"
  Thruster1/1(L1Vent) -> Bus Creator2/1  "L1Vent"
  Thruster1/2(L2Vent) -> Bus Creator2/2  "L2Vent"
  FeedPressure/1 -> Thruster1/2(FeedPressure)
  Constant/1 -> Switch/1
  Constant1/1 -> Switch/3
  Thruster1/4(thrusterData) -> XYZData/1  "A1TXYZ1"
  Data/1 -> Bus Selector/1
  Bus Selector/1 -> Thruster1/1(ValveAssign)  "<XYZValves>"
  Bus Selector/2 -> Thruster1/3(MainSwitch)  "<XYZSwitch>"
  Thruster1/3(Forces) -> XYZforces/1, Switch/2
  Switch/1 -> Bus Creator2/3  "Active1"
  Bus Creator2/1 -> Activitydata/1  "XYZ"

== system MultipleAgentsChoice_NoVR/StatePropagation/SatelliteControlAccel/Agent Body1/Actual Thruster response/Xthruster ==
  note: Tank pressure and thruster selection: must declare number of thrusters
  note: NB:-Agent has no knowledge of red blocks
      |             -Blue blocks prescribed by agent
  FeedPressure : Inport  OutDataType=sfix(16)  OutScaling=2^0
  ForceRequest : Inport  Port=2  OutDataType=sfix(16)  OutScaling=2^0
  Data : Inport  Port=3  OutDataType=sfix(16)  OutScaling=2^0
  Bus Creator2 : BusCreator  Inputs=3
  Bus Selector : BusSelector  OutputSignals=XValves1,XSwitch1
  Constant : Constant  OutDataType=sfix(16)  OutScaling=2^0
  Constant1 : Constant  Value=0  OutDataType=sfix(16)  OutScaling=2^0
  Switch : Switch  Criteria=u2 ~= 0
  Thruster1 : Subsystem
  XData : Outport  OutDataType=sfix(16)  OutScaling=2^0
  Xforces : Outport  Port=2  OutDataType=sfix(16)  OutScaling=2^0
  ActivityData : Outport  Port=3  OutDataType=sfix(16)  OutScaling=2^0
  wires:
  Bus Creator2/1 -> ActivityData/1
  Switch/1 -> Bus Creator2/3  "Active1"
  Thruster1/3(Forces) -> Xforces/1, Switch/2
  Bus Selector/2 -> Thruster1/3(MainSwitch)  "<XSwitch1>"
  Bus Selector/1 -> Thruster1/1(ValveAssign)  "<XValves1>"
  Data/1 -> Bus Selector/1
  Thruster1/4(ThrusterData) -> XData/1
  Constant1/1 -> Switch/3
  Constant/1 -> Switch/1
  FeedPressure/1 -> Thruster1/2(FeedPressure)
  Thruster1/2(L2Vent) -> Bus Creator2/2  "L2Vent"
  Thruster1/1(L1Vent) -> Bus Creator2/1  "L1Vent"
  ForceRequest/1 -> Thruster1/4(ForceRequest)  "Xforces"

== system MultipleAgentsChoice_NoVR/StatePropagation/SatelliteControlAccel/Agent Body1/Actual Thruster response/Ythruster1 ==
  note: NB:-Agent has no knowledge of red blocks
      |             -Blue blocks prescribed by agent
  note: Tank pressure and thruster selection: must declare number of thrusters
  FeedPressure : Inport  OutDataType=sfix(16)  OutScaling=2^0
  ForceRequest : Inport  Port=2  OutDataType=sfix(16)  OutScaling=2^0
  Data : Inport  Port=3  OutDataType=sfix(16)  OutScaling=2^0
  Bus Creator2 : BusCreator  Inputs=3
  Bus Selector : BusSelector  OutputSignals=YValves,YSwitch
  Constant : Constant  OutDataType=sfix(16)  OutScaling=2^0
  Constant1 : Constant  Value=0  OutDataType=sfix(16)  OutScaling=2^0
  Switch : Switch  Criteria=u2 ~= 0
  Thruster1 : Subsystem
  YData : Outport  OutDataType=sfix(16)  OutScaling=2^0
  Yforces : Outport  Port=2  OutDataType=sfix(16)  OutScaling=2^0
  ActivityData : Outport  Port=3  OutDataType=sfix(16)  OutScaling=2^0
  wires:
  ForceRequest/1 -> Thruster1/4(ForceRequest)  "Yforces"
  Thruster1/1(L1Vent) -> Bus Creator2/1  "L1Vent"
  Thruster1/2(L2Vent) -> Bus Creator2/2  "L2Vent"
  [ValveAssign1] -> Thruster1/1(ValveAssign)
  [MainSwitch1] -> Thruster1/3(MainSwitch)
  FeedPressure/1 -> Thruster1/2(FeedPressure)
  Constant/1 -> Switch/1
  Constant1/1 -> Switch/3
  Thruster1/4(thrusterData) -> YData/1  "A1TY1"
  Data/1 -> Bus Selector/1
  Bus Selector/1 -> [ValveAssign1]  "<YValves>"
  Bus Selector/2 -> [MainSwitch1]  "<YSwitch>"
  Thruster1/3(Forces) -> Yforces/1, Switch/2
  Switch/1 -> Bus Creator2/3  "Active1"
  Bus Creator2/1 -> ActivityData/1

== system MultipleAgentsChoice_NoVR/StatePropagation/SatelliteControlAccel/Agent Body1/Actual Thruster response/Zthruster1 ==
  note: Tank pressure and thruster selection: must declare number of thrusters
  note: NB:-Agent has no knowledge of red blocks
      |             -Blue blocks prescribed by agent
  FeedPressure : Inport  OutDataType=sfix(16)  OutScaling=2^0
  ForceRequest : Inport  Port=2  OutDataType=sfix(16)  OutScaling=2^0
  Data : Inport  Port=3  OutDataType=sfix(16)  OutScaling=2^0
  Reliability : Inport  Port=4  OutDataType=sfix(16)  OutScaling=2^0
  BrokenLine : Inport  Port=5  OutDataType=sfix(16)  OutScaling=2^0
  Bus Creator2 : BusCreator  Inputs=3
  Bus Selector : BusSelector  OutputSignals=ZValves,ZSwitch
  Constant : Constant  OutDataType=sfix(16)  OutScaling=2^0
  Constant1 : Constant  Value=0  OutDataType=sfix(16)  OutScaling=2^0
  Switch : Switch  Criteria=u2 ~= 0
  Thruster1 : Subsystem
  ZData : Outport  OutDataType=sfix(16)  OutScaling=2^0
  Zforces : Outport  Port=2  OutDataType=sfix(16)  OutScaling=2^0
  Activitydata : Outport  Port=3  OutDataType=sfix(16)  OutScaling=2^0
  wires:
  Reliability/1 -> Thruster1/5(Reliability)
  Bus Creator2/1 -> Activitydata/1
  Switch/1 -> Bus Creator2/3  "Active1"
  Thruster1/3(Forces) -> Switch/2, Zforces/1
  Bus Selector/2 -> Thruster1/3(MainSwitch)  "<ZSwitch>"
  Bus Selector/1 -> Thruster1/1(ValveAssign)  "<ZValves>"
  Data/1 -> Bus Selector/1
  Thruster1/4(thrusterData) -> ZData/1  "A1TZ1"
  Constant1/1 -> Switch/3
  Constant/1 -> Switch/1
  FeedPressure/1 -> Thruster1/2(FeedPressure)
  Thruster1/2(L2Vent) -> Bus Creator2/2  "L2Vent"
  Thruster1/1(L1Vent) -> Bus Creator2/1  "L1Vent"
  ForceRequest/1 -> Thruster1/4(ForceRequest)  "Zforces"
  BrokenLine/1 -> Thruster1/6(BrokenLine)

== system MultipleAgentsChoice_NoVR/StatePropagation/SatelliteControlAccel/Agent Body2/Actual Thruster response/PressureTank ==
  NumThrusters : Inport  OutDataType=sfix(16)  OutScaling=2^0
  GroupVentData : Inport  Port=2  OutDataType=sfix(16)  OutScaling=2^0
  Clock : Clock
      settings: Decimation=10
  Display : Display
  DropRate : MATLABFcn  MATLABFcn=DropRate_multi  OutputDimensions=1
  Integrator : Integrator  InitialConditionSource=external
  Mux : Mux  Inputs=2
  Start : Constant  Value=0  OutDataType=sfix(16)  OutScaling=2^0
  StartPressure : Constant  Value=100  OutDataType=sfix(16)  OutScaling=2^0
  Switch1 : Switch
  TankPressure : Outport  OutDataType=sfix(16)  OutScaling=2^0
  wires:
  StartPressure/1 -> Integrator/2
  Integrator/1 -> TankPressure/1, Display/1
  Start/1 -> Switch1/3
  Clock/1 -> Switch1/2
  Switch1/1 -> Integrator/1
  GroupVentData/1 -> Mux/2
  NumThrusters/1 -> Mux/1
  Mux/1 -> DropRate/1
  DropRate/1 -> Switch1/1

== system MultipleAgentsChoice_NoVR/StatePropagation/SatelliteControlAccel/Agent Body2/Actual Thruster response/XYZthruster ==
  note: Tank pressure and thruster selection: must declare number of thrusters
  note: NB:-Agent has no knowledge of red blocks
      |             -Blue blocks prescribed by agent
  FeedPressure : Inport  OutDataType=sfix(16)  OutScaling=2^0
  ForceRequest : Inport  Port=2  OutDataType=sfix(16)  OutScaling=2^0
  Data : Inport  Port=3  OutDataType=sfix(16)  OutScaling=2^0
  Bus Creator2 : BusCreator  Inputs=3
  Bus Selector : BusSelector  OutputSignals=XYZValves,XYZSwitch
  Constant : Constant  OutDataType=sfix(16)  OutScaling=2^0
  Constant1 : Constant  Value=0  OutDataType=sfix(16)  OutScaling=2^0
  Switch : Switch  Criteria=u2 ~= 0
  Thruster1 : Subsystem
  XYZData : Outport  OutDataType=sfix(16)  OutScaling=2^0
  XYZforces : Outport  Port=2  OutDataType=sfix(16)  OutScaling=2^0
  Activitydata : Outport  Port=3  OutDataType=sfix(16)  OutScaling=2^0
  wires:
  Bus Creator2/1 -> Activitydata/1  "XYZ"
  Switch/1 -> Bus Creator2/3  "Active1"
  Thruster1/3(Forces) -> Switch/2, XYZforces/1
  Bus Selector/2 -> Thruster1/3(MainSwitch)  "<XYZSwitch>"
  Bus Selector/1 -> Thruster1/1(ValveAssign)  "<XYZValves>"
  Data/1 -> Bus Selector/1
  Thruster1/4(thrusterData) -> XYZData/1
  Constant1/1 -> Switch/3
  Constant/1 -> Switch/1
  FeedPressure/1 -> Thruster1/2(FeedPressure)
  Thruster1/2(L2Vent) -> Bus Creator2/2  "L2Vent"
  Thruster1/1(L1Vent) -> Bus Creator2/1  "L1Vent"
  ForceRequest/1 -> Thruster1/4(ForceRequest)  "XYZforces"

== system MultipleAgentsChoice_NoVR/StatePropagation/SatelliteControlAccel/Agent Body2/Actual Thruster response/Xthruster ==
  note: NB:-Agent has no knowledge of red blocks
      |             -Blue blocks prescribed by agent
  note: Tank pressure and thruster selection: must declare number of thrusters
  FeedPressure : Inport  OutDataType=sfix(16)  OutScaling=2^0
  ForceRequest : Inport  Port=2  OutDataType=sfix(16)  OutScaling=2^0
  Data : Inport  Port=3  OutDataType=sfix(16)  OutScaling=2^0
  Bus Creator2 : BusCreator  Inputs=3
  Bus Selector : BusSelector  OutputSignals=XValves1,XSwitch1
  Constant : Constant  OutDataType=sfix(16)  OutScaling=2^0
  Constant1 : Constant  Value=0  OutDataType=sfix(16)  OutScaling=2^0
  Switch : Switch  Criteria=u2 ~= 0
  Thruster1 : Subsystem
  XData : Outport  OutDataType=sfix(16)  OutScaling=2^0
  Xforces : Outport  Port=2  OutDataType=sfix(16)  OutScaling=2^0
  ActivityData : Outport  Port=3  OutDataType=sfix(16)  OutScaling=2^0
  wires:
  ForceRequest/1 -> Thruster1/4(ForceRequest)  "Xforces"
  Thruster1/1(L1Vent) -> Bus Creator2/1  "L1Vent"
  Thruster1/2(L2Vent) -> Bus Creator2/2  "L2Vent"
  FeedPressure/1 -> Thruster1/2(FeedPressure)
  Constant/1 -> Switch/1
  Constant1/1 -> Switch/3
  Thruster1/4(ThrusterData) -> XData/1  "A2TX"
  Data/1 -> Bus Selector/1
  Bus Selector/1 -> Thruster1/1(ValveAssign)  "<XValves1>"
  Bus Selector/2 -> Thruster1/3(MainSwitch)  "<XSwitch1>"
  Thruster1/3(Forces) -> Switch/2, Xforces/1
  Switch/1 -> Bus Creator2/3  "Active1"
  Bus Creator2/1 -> ActivityData/1

== system MultipleAgentsChoice_NoVR/StatePropagation/SatelliteControlAccel/Agent Body2/Actual Thruster response/Ythruster1 ==
  note: Tank pressure and thruster selection: must declare number of thrusters
  note: NB:-Agent has no knowledge of red blocks
      |             -Blue blocks prescribed by agent
  FeedPressure : Inport  OutDataType=sfix(16)  OutScaling=2^0
  ForceRequest : Inport  Port=2  OutDataType=sfix(16)  OutScaling=2^0
  Data : Inport  Port=3  OutDataType=sfix(16)  OutScaling=2^0
  Bus Creator2 : BusCreator  Inputs=3
  Bus Selector : BusSelector  OutputSignals=YValves,YSwitch
  Constant : Constant  OutDataType=sfix(16)  OutScaling=2^0
  Constant1 : Constant  Value=0  OutDataType=sfix(16)  OutScaling=2^0
  Switch : Switch  Criteria=u2 ~= 0
  Thruster1 : Subsystem
  YData : Outport  OutDataType=sfix(16)  OutScaling=2^0
  Yforces : Outport  Port=2  OutDataType=sfix(16)  OutScaling=2^0
  ActivityData : Outport  Port=3  OutDataType=sfix(16)  OutScaling=2^0
  wires:
  Bus Creator2/1 -> ActivityData/1
  Switch/1 -> Bus Creator2/3  "Active1"
  Thruster1/3(Forces) -> Switch/2, Yforces/1
  Bus Selector/2 -> [MainSwitch1]  "<YSwitch>"
  Bus Selector/1 -> [ValveAssign1]  "<YValves>"
  Data/1 -> Bus Selector/1
  Thruster1/4(thrusterData) -> YData/1  "A2TY"
  Constant1/1 -> Switch/3
  Constant/1 -> Switch/1
  FeedPressure/1 -> Thruster1/2(FeedPressure)
  [MainSwitch1] -> Thruster1/3(MainSwitch)
  [ValveAssign1] -> Thruster1/1(ValveAssign)
  Thruster1/2(L2Vent) -> Bus Creator2/2  "L2Vent"
  Thruster1/1(L1Vent) -> Bus Creator2/1  "L1Vent"
  ForceRequest/1 -> Thruster1/4(ForceRequest)  "Yforces"

== system MultipleAgentsChoice_NoVR/StatePropagation/SatelliteControlAccel/Agent Body2/Actual Thruster response/Zthruster1 ==
  note: NB:-Agent has no knowledge of red blocks
      |             -Blue blocks prescribed by agent
  note: Tank pressure and thruster selection: must declare number of thrusters
  FeedPressure : Inport  OutDataType=sfix(16)  OutScaling=2^0
  ForceRequest : Inport  Port=2  OutDataType=sfix(16)  OutScaling=2^0
  Data : Inport  Port=3  OutDataType=sfix(16)  OutScaling=2^0
  Reliability : Inport  Port=4  OutDataType=sfix(16)  OutScaling=2^0
  BrokenLine : Inport  Port=5  OutDataType=sfix(16)  OutScaling=2^0
  Bus Creator2 : BusCreator  Inputs=3
  Bus Selector : BusSelector  OutputSignals=ZValves,ZSwitch
  Constant : Constant  OutDataType=sfix(16)  OutScaling=2^0
  Constant1 : Constant  Value=0  OutDataType=sfix(16)  OutScaling=2^0
  Switch : Switch  Criteria=u2 ~= 0
  Thruster1 : Subsystem
  ZData : Outport  OutDataType=sfix(16)  OutScaling=2^0
  Zforces : Outport  Port=2  OutDataType=sfix(16)  OutScaling=2^0
  Activitydata : Outport  Port=3  OutDataType=sfix(16)  OutScaling=2^0
  wires:
  ForceRequest/1 -> Thruster1/4(ForceRequest)  "Zforces"
  Thruster1/1(L1Vent) -> Bus Creator2/1  "L1Vent"
  Thruster1/2(L2Vent) -> Bus Creator2/2  "L2Vent"
  FeedPressure/1 -> Thruster1/2(FeedPressure)
  Constant/1 -> Switch/1
  Constant1/1 -> Switch/3
  Thruster1/4(thrusterData) -> ZData/1  "A2TZ"
  Data/1 -> Bus Selector/1
  Bus Selector/1 -> Thruster1/1(ValveAssign)  "<ZValves>"
  Bus Selector/2 -> Thruster1/3(MainSwitch)  "<ZSwitch>"
  Thruster1/3(Forces) -> Zforces/1, Switch/2
  Switch/1 -> Bus Creator2/3  "Active1"
  Bus Creator2/1 -> Activitydata/1
  Reliability/1 -> Thruster1/5(Reliability)
  BrokenLine/1 -> Thruster1/6(BrokenLine)

== system MultipleAgentsChoice_NoVR/StatePropagation/SatelliteControlAccel/Agent Body3/Actual Thruster response/PressureTank ==
  NumThrusters : Inport  OutDataType=sfix(16)  OutScaling=2^0
  GroupVentData : Inport  Port=2  OutDataType=sfix(16)  OutScaling=2^0
  Clock : Clock
      settings: Decimation=10
  Display : Display
  DropRate : MATLABFcn  MATLABFcn=DropRate_multi  OutputDimensions=1
  Integrator : Integrator  InitialConditionSource=external
  Mux : Mux  Inputs=2
  Start : Constant  Value=0  OutDataType=sfix(16)  OutScaling=2^0
  StartPressure : Constant  Value=100  OutDataType=sfix(16)  OutScaling=2^0
  Switch1 : Switch
  TankPressure : Outport  OutDataType=sfix(16)  OutScaling=2^0
  wires:
  StartPressure/1 -> Integrator/2
  Integrator/1 -> TankPressure/1, Display/1
  Start/1 -> Switch1/3
  Clock/1 -> Switch1/2
  Switch1/1 -> Integrator/1
  GroupVentData/1 -> Mux/2
  NumThrusters/1 -> Mux/1
  Mux/1 -> DropRate/1
  DropRate/1 -> Switch1/1

== system MultipleAgentsChoice_NoVR/StatePropagation/SatelliteControlAccel/Agent Body3/Actual Thruster response/XYZthruster ==
  note: Tank pressure and thruster selection: must declare number of thrusters
  note: NB:-Agent has no knowledge of red blocks
      |             -Blue blocks prescribed by agent
  FeedPressure : Inport  OutDataType=sfix(16)  OutScaling=2^0
  ForceRequest : Inport  Port=2  OutDataType=sfix(16)  OutScaling=2^0
  Data : Inport  Port=3  OutDataType=sfix(16)  OutScaling=2^0
  Bus Creator2 : BusCreator  Inputs=3
  Bus Selector : BusSelector  OutputSignals=XYZValves,XYZSwitch
  Constant : Constant  OutDataType=sfix(16)  OutScaling=2^0
  Constant1 : Constant  Value=0  OutDataType=sfix(16)  OutScaling=2^0
  Switch : Switch  Criteria=u2 ~= 0
  Thruster1 : Subsystem
  XYZData : Outport  OutDataType=sfix(16)  OutScaling=2^0
  XYZforces : Outport  Port=2  OutDataType=sfix(16)  OutScaling=2^0
  Activitydata : Outport  Port=3  OutDataType=sfix(16)  OutScaling=2^0
  wires:
  Bus Creator2/1 -> Activitydata/1  "XYZ"
  Switch/1 -> Bus Creator2/3  "Active1"
  Thruster1/3(Forces) -> Switch/2, XYZforces/1
  Bus Selector/2 -> Thruster1/3(MainSwitch)  "<XYZSwitch>"
  Bus Selector/1 -> Thruster1/1(ValveAssign)  "<XYZValves>"
  Data/1 -> Bus Selector/1
  Thruster1/4(thrusterData) -> XYZData/1  "A3TXYZ"
  Constant1/1 -> Switch/3
  Constant/1 -> Switch/1
  FeedPressure/1 -> Thruster1/2(FeedPressure)
  Thruster1/2(L2Vent) -> Bus Creator2/2  "L2Vent"
  Thruster1/1(L1Vent) -> Bus Creator2/1  "L1Vent"
  ForceRequest/1 -> Thruster1/4(ForceRequest)  "XYZforces"

== system MultipleAgentsChoice_NoVR/StatePropagation/SatelliteControlAccel/Agent Body3/Actual Thruster response/Xthruster ==
  note: NB:-Agent has no knowledge of red blocks
      |             -Blue blocks prescribed by agent
  note: Tank pressure and thruster selection: must declare number of thrusters
  FeedPressure : Inport  OutDataType=sfix(16)  OutScaling=2^0
  ForceRequest : Inport  Port=2  OutDataType=sfix(16)  OutScaling=2^0
  Data : Inport  Port=3  OutDataType=sfix(16)  OutScaling=2^0
  Bus Creator2 : BusCreator  Inputs=3
  Bus Selector : BusSelector  OutputSignals=XValves1,XSwitch1
  Constant : Constant  OutDataType=sfix(16)  OutScaling=2^0
  Constant1 : Constant  Value=0  OutDataType=sfix(16)  OutScaling=2^0
  Switch : Switch  Criteria=u2 ~= 0
  Thruster1 : Subsystem
  XData : Outport  OutDataType=sfix(16)  OutScaling=2^0
  Xforces : Outport  Port=2  OutDataType=sfix(16)  OutScaling=2^0
  ActivityData : Outport  Port=3  OutDataType=sfix(16)  OutScaling=2^0
  wires:
  ForceRequest/1 -> Thruster1/4(ForceRequest)  "Xforces"
  Thruster1/1(L1Vent) -> Bus Creator2/1  "L1Vent"
  Thruster1/2(L2Vent) -> Bus Creator2/2  "L2Vent"
  FeedPressure/1 -> Thruster1/2(FeedPressure)
  Constant/1 -> Switch/1
  Constant1/1 -> Switch/3
  Thruster1/4(ThrusterData) -> XData/1  "A3TX"
  Data/1 -> Bus Selector/1
  Bus Selector/1 -> Thruster1/1(ValveAssign)  "<XValves1>"
  Bus Selector/2 -> Thruster1/3(MainSwitch)  "<XSwitch1>"
  Thruster1/3(Forces) -> Switch/2, Xforces/1
  Switch/1 -> Bus Creator2/3  "Active1"
  Bus Creator2/1 -> ActivityData/1

== system MultipleAgentsChoice_NoVR/StatePropagation/SatelliteControlAccel/Agent Body3/Actual Thruster response/Ythruster1 ==
  note: Tank pressure and thruster selection: must declare number of thrusters
  note: NB:-Agent has no knowledge of red blocks
      |             -Blue blocks prescribed by agent
  FeedPressure : Inport  OutDataType=sfix(16)  OutScaling=2^0
  ForceRequest : Inport  Port=2  OutDataType=sfix(16)  OutScaling=2^0
  Data : Inport  Port=3  OutDataType=sfix(16)  OutScaling=2^0
  Bus Creator2 : BusCreator  Inputs=3
  Bus Selector : BusSelector  OutputSignals=YValves,YSwitch
  Constant : Constant  OutDataType=sfix(16)  OutScaling=2^0
  Constant1 : Constant  Value=0  OutDataType=sfix(16)  OutScaling=2^0
  Switch : Switch  Criteria=u2 ~= 0
  Thruster1 : Subsystem
  YData : Outport  OutDataType=sfix(16)  OutScaling=2^0
  Yforces : Outport  Port=2  OutDataType=sfix(16)  OutScaling=2^0
  ActivityData : Outport  Port=3  OutDataType=sfix(16)  OutScaling=2^0
  wires:
  Bus Creator2/1 -> ActivityData/1
  Switch/1 -> Bus Creator2/3  "Active1"
  Thruster1/3(Forces) -> Switch/2, Yforces/1
  Bus Selector/2 -> [MainSwitch1]  "<YSwitch>"
  Bus Selector/1 -> [ValveAssign1]  "<YValves>"
  Data/1 -> Bus Selector/1
  Thruster1/4(thrusterData) -> YData/1  "A3TY"
  Constant1/1 -> Switch/3
  Constant/1 -> Switch/1
  FeedPressure/1 -> Thruster1/2(FeedPressure)
  [MainSwitch1] -> Thruster1/3(MainSwitch)
  [ValveAssign1] -> Thruster1/1(ValveAssign)
  Thruster1/2(L2Vent) -> Bus Creator2/2  "L2Vent"
  Thruster1/1(L1Vent) -> Bus Creator2/1  "L1Vent"
  ForceRequest/1 -> Thruster1/4(ForceRequest)  "Yforces"
